simulink model "switchTest"  (Simulink 7.9)
settings: Solver=ode45  StartTime=0.0  StopTime=60  MaxStep=0.001  RelTol=1e-3
settings Model: Creator=root  LastModifiedBy=root

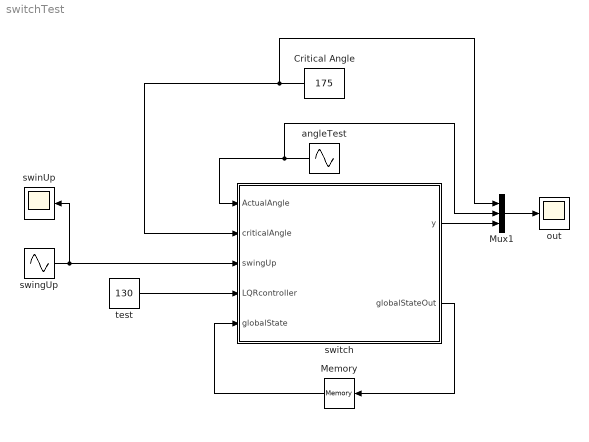
== system switchTest ==
  Critical Angle : Constant  Value=175
  Memory : Memory
  Mux1 : Mux  Inputs=3
  angleTest : Sin  Amplitude=20  Bias=160  Frequency=0.1
  out : Scope
      settings: YMin=115  YMax=180
  swinUp : Scope
  swingUp : Sin  Amplitude=2  Bias=120  Frequency=10
  switch : MATLAB Function  TreatAsAtomicUnit=on
  test : Constant  Value=130
  wires:
  swingUp/1 -> switch/3(swingUp), swinUp/1
  Critical Angle/1 -> switch/2(criticalAngle), Mux1/1
  test/1 -> switch/4(LQRcontroller)
  angleTest/1 -> switch/1(ActualAngle), Mux1/2
  Mux1/1 -> out/1
  switch/2(globalStateOut) -> Memory/1
  Memory/1 -> switch/5(globalState)
  switch/1(y) -> Mux1/3

== matlab function switch ==
  data: y output double; ActualAngle input double; criticalAngle input double; swingUp input double; LQRcontroller input double; globalState input double; globalStateOut output double
function [y, globalStateOut] = controllerSwitch(ActualAngle, criticalAngle, swingUp, LQRcontroller, globalState)
%function y = fcn(swingUp, LQRcontroller, globalState)
%
if (ActualAngle < criticalAngle && globalState == 0)
    y = swingUp;
    globalStateOut = 0;
else% if (ActualAngle >= criticalAngle || globalState > 1)
    y = LQRcontroller;
    globalStateOut = 1;
end

end
